simulink model "random_b"  (Simulink 7.1)
settings: Solver=ode45  StartTime=0.0  StopTime=60.0  RelTol=1e-3
settings Model: Creator=Usuario  LastModifiedBy=Usuario  BufferReuse=off
settings OptimizationCC: OptimizeBlockIOStorage=off  BufferReuse=off  ExpressionFolding=off  LocalBlockOutputs=off

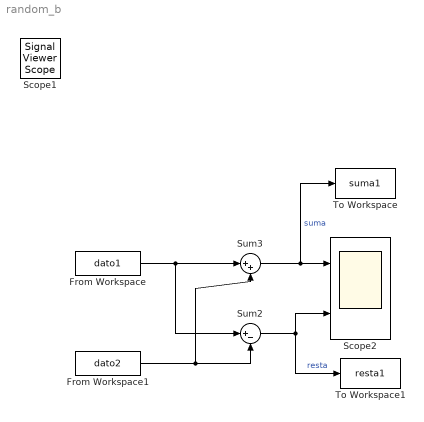
== system random_b ==
  From Workspace : FromWorkspace  VariableName=dato1  SampleTime=0.1
  From Workspace1 : FromWorkspace  VariableName=dato2  SampleTime=0.1
  Scope2 : Scope  NumInputPorts=2
      settings: YMin=-5~-5  YMax=5~5  SaveName=ScopeData2
  Sum2 : Sum  Inputs=|+-  OutDataType=sfix(16)  OutScaling=2^0
  Sum3 : Sum  Inputs=|++  OutDataType=sfix(16)  OutScaling=2^0
  To Workspace : ToWorkspace  VariableName=suma1  SampleTime=-1  SaveFormat=Structure
  To Workspace1 : ToWorkspace  VariableName=resta1  SampleTime=-1  SaveFormat=Structure
  Scope1 : SignalViewerScope  IOType=viewer  RefreshTime=0.035000
  wires:
  From Workspace/1 -> Sum3/1, Sum2/1
  From Workspace1/1 -> Sum2/2, Sum3/2
  Sum3/1 -> Scope2/1, To Workspace/1  "suma"
  Sum2/1 -> Scope2/2, To Workspace1/1  "resta"
